simulink model "mainWOLVESnRABBIT"  (R2024b)
settings: Solver=VariableStepAuto  StartTime=0.0  StopTime=240  RelTol=1e-3
settings Model: Creator=z1186362
settings RTWCC: GPUComputeCapability=3.5

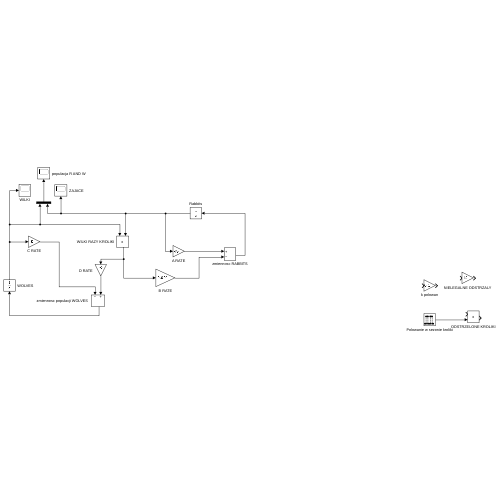
[thumbnail: Simulink's stored preview of the top-level diagram]
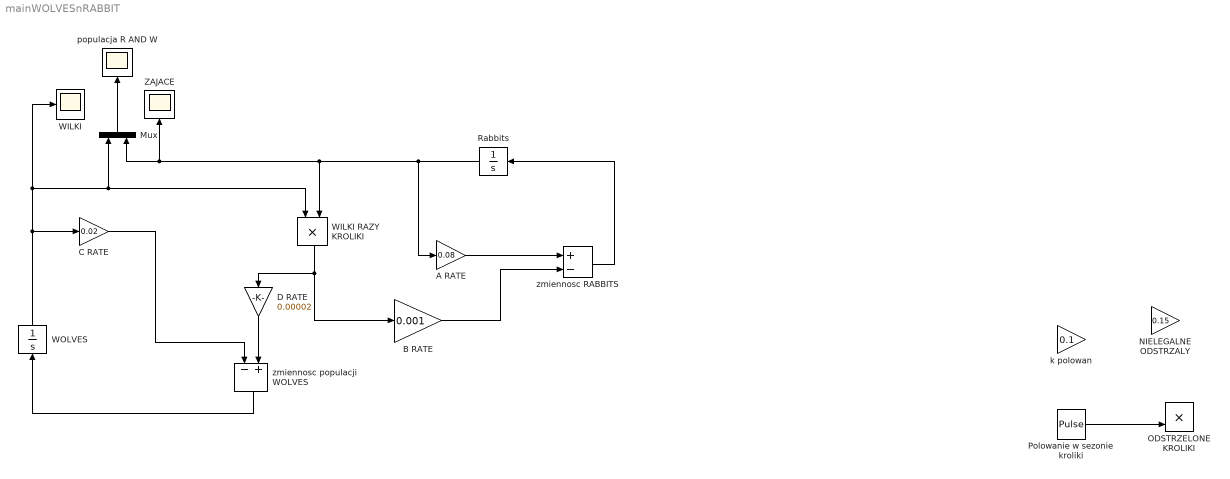
== system mainWOLVESnRABBIT ==
  A RATE : Gain  Gain=0.08
  B RATE : Gain  Gain=0.001
  C RATE : Gain  Gain=0.02
  D RATE : Gain  Gain=0.00002
  Mux : Mux  Inputs=2
  NIELEGALNE ODSTRZALY : Gain  Gain=0.15
  ODSTRZELONE KROLIKI : Product
  Polowanie w sezonie kroliki : DiscretePulseGenerator  Amplitude=0.18  Period=6
  Rabbits : Integrator  InitialCondition=1000
  WILKI : Scope
  WILKI RAZY KROLIKI : Product
  WOLVES : Integrator  InitialCondition=40
  ZAJACE : Scope
  k polowan : Gain  Gain=0.1
  populacja R AND W : Scope
  zmiennosc RABBITS : Sum  Inputs=+-
  "zmiennosc populacji WOLVES " : Sum  Inputs=-+
  wires:
  zmiennosc RABBITS/1 -> Rabbits/1
  "zmiennosc populacji WOLVES "/1 -> WOLVES/1
  Rabbits/1 -> A RATE/1, WILKI RAZY KROLIKI/2, ZAJACE/1, Mux/2
  A RATE/1 -> zmiennosc RABBITS/1
  Polowanie w sezonie kroliki/1 -> ODSTRZELONE KROLIKI/2
  WOLVES/1 -> WILKI/1, Mux/1, WILKI RAZY KROLIKI/1, C RATE/1
  WILKI RAZY KROLIKI/1 -> B RATE/1, D RATE/1
  Mux/1 -> populacja R AND W/1
  C RATE/1 -> "zmiennosc populacji WOLVES "/1
  D RATE/1 -> "zmiennosc populacji WOLVES "/2
  B RATE/1 -> zmiennosc RABBITS/2
